simulink model "gm_broadwayIPC_2024b_interface"  (R2024b)
settings: Solver=FixedStepDiscrete  StartTime=0.0  StopTime=2  RelTol=1e-3  EnableMultiTasking=on
undefined symbols (not defined in the file or in its folder): gray
libraries: hdlsllib x20, visionhdlio x6, visionsources x2
Description:
  | Sobel Edge Detection Using the MATLAB(R) Function Block
  | This example shows how to use HDL Coder(TM) to check,
  | generate, and verify HDL code for a Sobel Edge Detection
  | block built using the MATLAB Function block.
settings Model: Creator=The MathWorks, Inc.  LastModifiedBy=Chris
settings SolverCC: AlgebraicLoopSolver=TrustRegion  PositivePriorityOrder=on
settings DataIOCC: LimitDataPoints=on  SaveFormat=Array  SignalLogging=off  ReturnWorkspaceOutputs=off
settings OptimizationCC: BlockReduction=off  ConditionallyExecuteInputs=off  EnhancedBackFolding=on  PassReuseOutputArgsAs=Individual arguments  ExpressionDepthLimit=2147483647  ZeroExternalMemoryAtStartup=off  ZeroInternalMemoryAtStartup=off  InitFltsAndDblsToZero=on  EfficientMapNaN2IntZero=off  MaxStackSize=64  OptimizeBlockOrder=speed  DifferentSizesBufferReuse=on  OptimizationCustomize=off  EfficientTunableParamExpr=on
settings DebuggingCC: AlgebraicLoopMsg=error  SaveWithParameterizedLinksMsg=none  UnderspecifiedInitializationDetection=Classic  MergeDetectMultiDrivingBlocksExec=none  SignalResolutionControl=TryResolveAllWithWarning  SingleTaskRateTransMsg=error  IntegerOverflowMsg=none  ParameterPrecisionLossMsg=none  ParameterTunabilityLossMsg=error  FcnCallInpInsideContextMsg=warning  UnconnectedInputMsg=warning  UnconnectedOutputMsg=warning  UnconnectedLineMsg=warning  AllowSymbolicDim=off  StateNameClashWarn=warning  StrictBusMsg=ErrorOnBusTreatedAsVector  SFUnexpectedBacktrackingDiag=warning  SFNoUnconditionalDefaultTransitionDiag=warning  SFExecutionAtInitializationDiag=none  IntegerSaturationMsg=none  ArithmeticOperatorsInVariantConditions=warning
settings HardwareCC: ProdBitPerPointer=32  ProdBitPerSizeT=32  ProdBitPerPtrDiffT=32  ProdLargestAtomicInteger=Long  ProdLargestAtomicFloat=Double  ProdWordSize=32  ProdLongLongMode=on  ProdHWDeviceType=ARM Compatible->ARM Cortex-A (32-bit)  TargetHWDeviceType=32-bit Generic
settings ModelReferenceCC: EnableRefExpFcnMdlSchedulingChecks=on  ModelReferenceNumInstancesAllowed=Single  PropagateSignalLabelsOutOfModel=off
settings SFSimCC: SimUseLocalCustomCode=off  MATLABDynamicMemAlloc=off  CustomCodeUndefinedFunction=UseInterfaceOnly
settings RTWCC: Description=Embedded Coder  SystemTargetFile=ert.tlc  HardwareBoard=Xilinx Zynq-7000 based board  TLCOptions="-aInlineSetEventsForThisBaseRateFcn=TLC_FALSE -aSuppressMultiTaskScheduler=TLC_FALSE  -aRateBasedStepFcn=0"  TemplateMakefile=ert_default_tmf  RTWUseLocalCustomCode=off  Toolchain=Linaro AArch32 Linux v6.3.1  GPUComputeCapability=3.5  DLArmComputeVersion=19.05
settings CodeAppCC: ForceParamTrailComments=on  IgnoreCustomStorageClasses=off  OperatorAnnotations=on  SimulinkDataObjDesc=on  SFDataObjDesc=on  InsertBlockDesc=on
settings ERTTargetCC: InlinedParameterPlacement=Hierarchical
settings ConfigComp: CovMetricSettings=dw  CovSaveCumulativeToWorkspaceVar=on  CovSaveSingleToWorkspaceVar=on  CovExternalEMLEnable=off

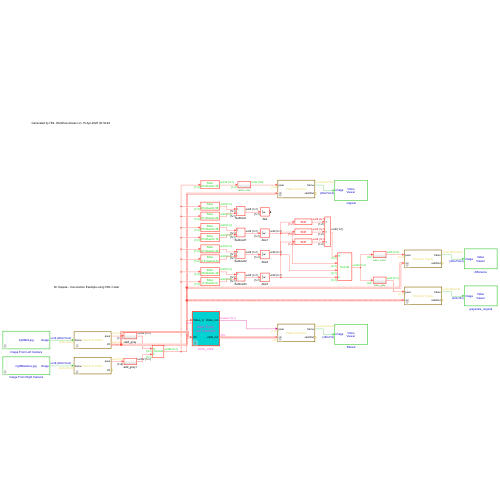
[thumbnail: Simulink's stored preview of the top-level diagram]
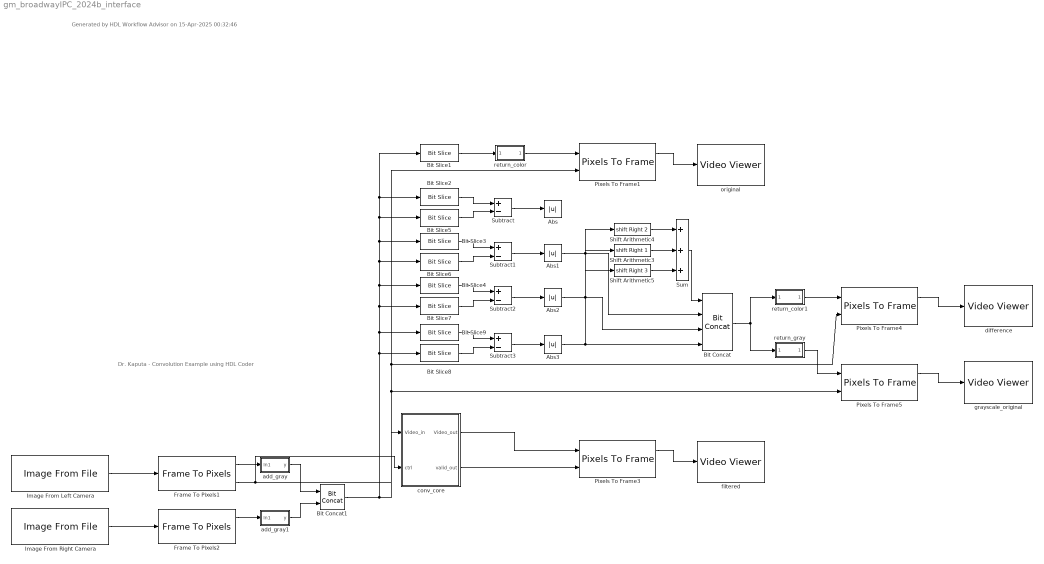
== system gm_broadwayIPC_2024b_interface ==
  note: Dr. Kaputa - Convolution Example using HDL Coder
  note: Generated by HDL Workflow Advisor on 15-Apr-2025 00:32:46
  Abs{,1..3} (4 alike) : Abs  OutDataTypeStr=uint8
  Bit Concat : hdlsllib/Logic and Bit Operations/Bit Concat  numInputs=4
  Bit Concat1 : hdlsllib/Logic and Bit Operations/Bit Concat  numInputs=2
  Bit Slice1 : hdlsllib/Logic and Bit Operations/Bit Slice  lidx=63  ridx=32
  Bit Slice2 : hdlsllib/Logic and Bit Operations/Bit Slice  lidx=63  ridx=56
  Bit Slice3 : hdlsllib/Logic and Bit Operations/Bit Slice  lidx=55  ridx=48
  Bit Slice4 : hdlsllib/Logic and Bit Operations/Bit Slice  lidx=47  ridx=40
  Bit Slice5 : hdlsllib/Logic and Bit Operations/Bit Slice  lidx=31  ridx=24
  Bit Slice6 : hdlsllib/Logic and Bit Operations/Bit Slice  lidx=23  ridx=16
  Bit Slice7 : hdlsllib/Logic and Bit Operations/Bit Slice  lidx=15  ridx=8
  Bit Slice8 : hdlsllib/Logic and Bit Operations/Bit Slice  lidx=7  ridx=0
  Bit Slice9 : hdlsllib/Logic and Bit Operations/Bit Slice  lidx=39  ridx=32
  Frame To Pixels1 : visionhdlio/Frame To Pixels  NumComponents=3  NumPixels=1  VideoFormat=Custom  ActivePixelsPerLine=R  ActiveVideoLines=C  TotalPixelsPerLine=R  TotalVideoLines=C  StartingActiveLine=1  FrontPorch=0  SampleTime=0  VideoFormatCache=Custom  ActivePixelsPerLineCache=R  ActiveVideoLinesCache=C  TotalPixelsPerLineCache=R  TotalVideoLinesCache=C  StartingActiveLineCache=1  FrontPorchCache=0
  Frame To Pixels2 : visionhdlio/Frame To Pixels  NumComponents=3  NumPixels=1  VideoFormat=Custom  ActivePixelsPerLine=R  ActiveVideoLines=C  TotalPixelsPerLine=R  TotalVideoLines=C  StartingActiveLine=1  FrontPorch=0  SampleTime=0  VideoFormatCache=Custom  ActivePixelsPerLineCache=R  ActiveVideoLinesCache=C  TotalPixelsPerLineCache=R  TotalVideoLinesCache=C  StartingActiveLineCache=1  FrontPorchCache=0
  Image From Left Camera : visionsources/Image From File  Tag=vipblks_nd  FileName=C:\Users\Chris\Documents\Repos\WiiSports\TennisTracker\BoradwaySimulink\rightBall.jpg  Ts=1  imagePorts=One multidimensional signal  OutPortLabels=R|G|B  ImageDataType=Inherit from input image  sdImageDataType=uint(8)  Signed=on  WordLength=16  FractionLengthMode=User-defined  FractionLength=15
  Image From Right Camera : visionsources/Image From File  Tag=vipblks_nd  FileName=C:\Users\Chris\Documents\Repos\WiiSports\TennisTracker\BoradwaySimulink\rightBaseline.jpg  Ts=1  imagePorts=One multidimensional signal  OutPortLabels=R|G|B  ImageDataType=Inherit from input image  sdImageDataType=uint(8)  Signed=on  WordLength=16  FractionLengthMode=User-defined  FractionLength=15
  Pixels To Frame1 : visionhdlio/Pixels To Frame  NumComponents=3  NumPixels=1  VideoFormat=Custom  ActivePixelsPerLine=R  ActiveVideoLines=C  TotalPixelsPerLine=R  TotalVideoLines=C  VideoFormatCache=Custom  ActivePixelsPerLineCache=R  ActiveVideoLinesCache=C  TotalPixelsPerLineCache=R  TotalVideoLinesCache=C
  Pixels To Frame3 : visionhdlio/Pixels To Frame  NumComponents=1  NumPixels=1  VideoFormat=Custom  ActivePixelsPerLine=R  ActiveVideoLines=C  TotalPixelsPerLine=R  TotalVideoLines=C  VideoFormatCache=Custom  ActivePixelsPerLineCache=R  ActiveVideoLinesCache=C  TotalPixelsPerLineCache=R  TotalVideoLinesCache=C
  Pixels To Frame4 : visionhdlio/Pixels To Frame  NumComponents=3  NumPixels=1  VideoFormat=Custom  ActivePixelsPerLine=R  ActiveVideoLines=C  TotalPixelsPerLine=R  TotalVideoLines=C  VideoFormatCache=Custom  ActivePixelsPerLineCache=R  ActiveVideoLinesCache=C  TotalPixelsPerLineCache=R  TotalVideoLinesCache=C
  Pixels To Frame5 : visionhdlio/Pixels To Frame  NumComponents=1  NumPixels=1  VideoFormat=Custom  ActivePixelsPerLine=R  ActiveVideoLines=C  TotalPixelsPerLine=R  TotalVideoLines=C  VideoFormatCache=Custom  ActivePixelsPerLineCache=R  ActiveVideoLinesCache=C  TotalPixelsPerLineCache=R  TotalVideoLinesCache=C
  Shift Arithmetic3 : ArithShift  BitShiftNumber=1  BitShiftDirection=Right
  Shift Arithmetic4 : ArithShift  BitShiftNumber=2  BitShiftDirection=Right
  Shift Arithmetic5 : ArithShift  BitShiftNumber=3  BitShiftDirection=Right
  Subtract{,1..3} (4 alike) : Sum  Inputs=+-
  Sum : Sum  Inputs=+++  OutDataTypeStr=uint8
  add_gray : Subsystem
  add_gray1 : Subsystem
  conv_core : Subsystem  TreatAsAtomicUnit=on  mask(AXI4-Lite/AXI4 Interface){}
      mask help:
      | This is an automatically generated subsystem block.
      | This contains the AXI interface blocks that communicate with the conv_core_ip IPCore generated from broadwayIPC_2024b/conv_core subsystem.
      mask Display: disp(sprintf('Xilinx Zynq \nAXI Interface'));
  difference : VideoViewer  FigPos=[994 1078 927 429]
  filtered : VideoViewer  colormapValue=gray(256)  FigPos=[66 1078 927 429]
  grayscale_original : VideoViewer  FigPos=[65 538 927 429]
  original : VideoViewer  FigPos=[995 538 927 429]
  return_color : Subsystem
  return_color1 : Subsystem
  return_gray : Subsystem
  wires:
  Bit Concat/1 -> return_color1/1(RGB), return_gray/1(RGB)
  Sum/1 -> Bit Concat/1
  Abs1/1 -> Bit Concat/2, Shift Arithmetic4/1
  Abs2/1 -> Bit Concat/3, Shift Arithmetic3/1
  Abs3/1 -> Bit Concat/4, Shift Arithmetic5/1
  Shift Arithmetic4/1 -> Sum/1
  Shift Arithmetic3/1 -> Sum/2
  Shift Arithmetic5/1 -> Sum/3
  return_gray/1(RGBVector) -> Pixels To Frame5/1
  Pixels To Frame5/1 -> grayscale_original/1
  Bit Slice8/1 -> Subtract3/2
  Bit Slice9/1 -> Subtract3/1
  Bit Slice7/1 -> Subtract2/2
  Bit Slice4/1 -> Subtract2/1
  Bit Slice6/1 -> Subtract1/2
  Bit Slice3/1 -> Subtract1/1
  Bit Slice5/1 -> Subtract/2
  Bit Slice2/1 -> Subtract/1
  Subtract3/1 -> Abs3/1
  Subtract2/1 -> Abs2/1
  Subtract1/1 -> Abs1/1
  return_color1/1(RGBVector) -> Pixels To Frame4/1
  Subtract/1 -> Abs/1
  Pixels To Frame4/1 -> difference/1
  Bit Slice1/1 -> return_color/1(RGB)
  add_gray1/1(y) -> Bit Concat1/2
  add_gray/1(y) -> Bit Concat1/1
  Frame To Pixels2/1 -> add_gray1/1(In1)
  Frame To Pixels1/2 -> Pixels To Frame4/2, Pixels To Frame1/2, Pixels To Frame5/2, conv_core/2(ctrl)
  Image From Right Camera/1 -> Frame To Pixels2/1
  conv_core/1(Video_out) -> Pixels To Frame3/1
  Bit Concat1/1 -> Bit Slice2/1, Bit Slice1/1, Bit Slice5/1, Bit Slice3/1, Bit Slice6/1, Bit Slice4/1, Bit Slice7/1, Bit Slice9/1, Bit Slice8/1, conv_core/1(Video_in)
  conv_core/2(valid_out) -> Pixels To Frame3/2
  Pixels To Frame3/1 -> filtered/1
  Frame To Pixels1/1 -> add_gray/1(In1)
  return_color/1(RGBVector) -> Pixels To Frame1/1
  Pixels To Frame1/1 -> original/1
  Image From Left Camera/1 -> Frame To Pixels1/1

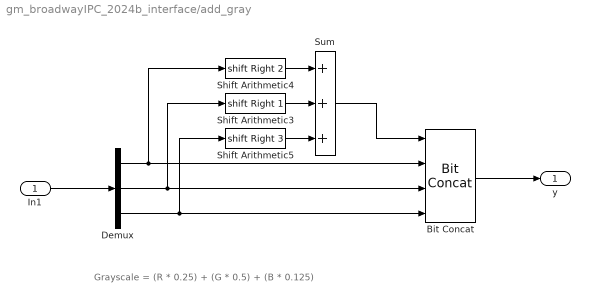
== system gm_broadwayIPC_2024b_interface/add_gray ==
  note: Grayscale = (R * 0.25) + (G * 0.5) + (B * 0.125)
  In1 : Inport
  Bit Concat : hdlsllib/Logic and Bit Operations/Bit Concat  numInputs=4
  Demux : Demux  Outputs=3
  Shift Arithmetic3 : ArithShift  BitShiftNumber=1  BitShiftDirection=Right
  Shift Arithmetic4 : ArithShift  BitShiftNumber=2  BitShiftDirection=Right
  Shift Arithmetic5 : ArithShift  BitShiftNumber=3  BitShiftDirection=Right
  Sum : Sum  Inputs=+++  OutDataTypeStr=uint8
  y : Outport
  wires:
  Shift Arithmetic5/1 -> Sum/3
  Shift Arithmetic3/1 -> Sum/2
  Shift Arithmetic4/1 -> Sum/1
  Sum/1 -> Bit Concat/1
  Demux/3 -> Bit Concat/4, Shift Arithmetic5/1
  Demux/1 -> Bit Concat/2, Shift Arithmetic4/1
  Demux/2 -> Bit Concat/3, Shift Arithmetic3/1
  In1/1 -> Demux/1
  Bit Concat/1 -> y/1

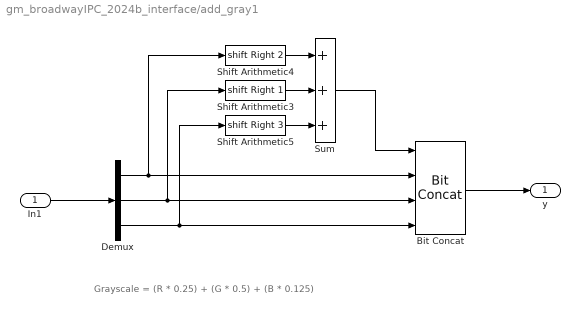
== system gm_broadwayIPC_2024b_interface/add_gray1 ==
  note: Grayscale = (R * 0.25) + (G * 0.5) + (B * 0.125)
  In1 : Inport
  Bit Concat : hdlsllib/Logic and Bit Operations/Bit Concat  numInputs=4
  Demux : Demux  Outputs=3
  Shift Arithmetic3 : ArithShift  BitShiftNumber=1  BitShiftDirection=Right
  Shift Arithmetic4 : ArithShift  BitShiftNumber=2  BitShiftDirection=Right
  Shift Arithmetic5 : ArithShift  BitShiftNumber=3  BitShiftDirection=Right
  Sum : Sum  Inputs=+++  OutDataTypeStr=uint8
  y : Outport
  wires:
  Sum/1 -> Bit Concat/1
  Shift Arithmetic5/1 -> Sum/3
  Shift Arithmetic3/1 -> Sum/2
  Shift Arithmetic4/1 -> Sum/1
  Demux/3 -> Bit Concat/4, Shift Arithmetic5/1
  Demux/1 -> Bit Concat/2, Shift Arithmetic4/1
  Demux/2 -> Bit Concat/3, Shift Arithmetic3/1
  In1/1 -> Demux/1
  Bit Concat/1 -> y/1

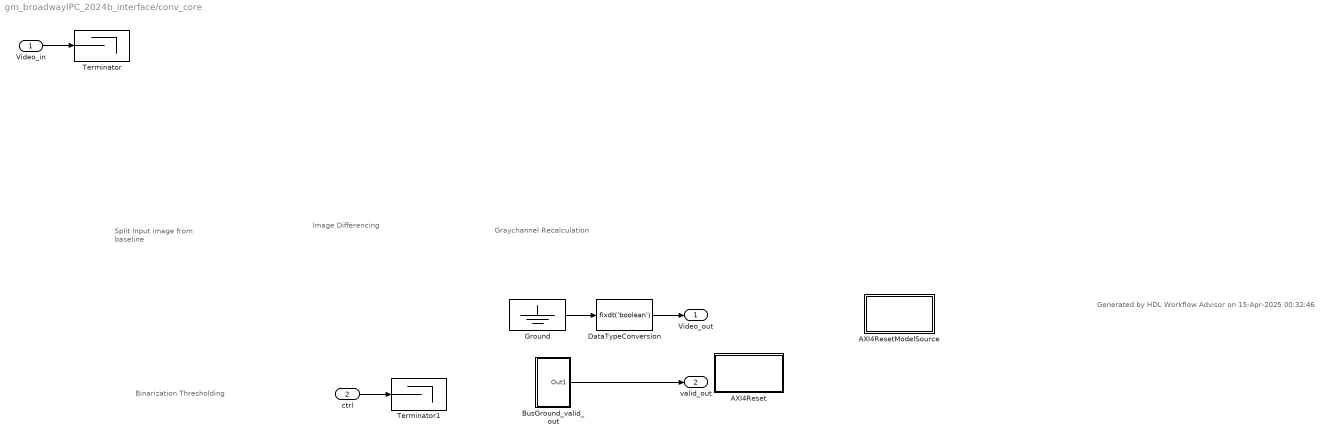
== system gm_broadwayIPC_2024b_interface/conv_core ==
  note: Binarization Thresholding
  note: Image
      | Differencing
  note: Split Input image
      | from baseline
  note: Graychannel Recalculation
  note: Generated by HDL Workflow Advisor on 15-Apr-2025 00:32:46
  Video_in : Inport
  ctrl : Inport  Port=2
  AXI4Reset : Subsystem  mask(System Start){ShowInLibBrowser=0}
      mask prompts: ShowInLibBrowser "Simulink:masks:CustCodeMaskParam1_MP"
      settings: CopyFcn=cccopyfcn(gcb)  OpenFcn=ccopenfcn('System Start Function')
      mask Help: eval('feval(''rtwprivate'',''rtwhelpview'',''rtw_sys_start_block'')');
      mask Display: disp('System\nStart');
  AXI4ResetModelSource : Subsystem  mask(Model Source){ShowInLibBrowser=0}
      mask prompts: ShowInLibBrowser "Simulink:masks:CustCodeMaskParam1_MP"
      settings: CopyFcn=cccopyfcn(gcb)  OpenFcn=ccopenfcn('Model Source')
      mask Help: eval('feval(''rtwprivate'',''rtwhelpview'',''rtw_model_source_block'')');
      mask Display: disp('Model\nSource');
  BusGround_valid_out : Subsystem
  DataTypeConversion : DataTypeConversion  OutDataTypeStr=fixdt('boolean')  ConvertRealWorld=Stored Integer (SI)  SaturateOnIntegerOverflow=off  RndMeth=Floor
  Ground : Ground
  Terminator : Terminator
  Terminator1 : Terminator
  Video_out : Outport  VectorParamsAs1DForOutWhenUnconnected=off
  valid_out : Outport  Port=2  VectorParamsAs1DForOutWhenUnconnected=off
  wires:
  Video_in/1 -> Terminator/1
  ctrl/1 -> Terminator1/1
  DataTypeConversion/1 -> Video_out/1
  Ground/1 -> DataTypeConversion/1
  BusGround_valid_out/1(Out1) -> valid_out/1

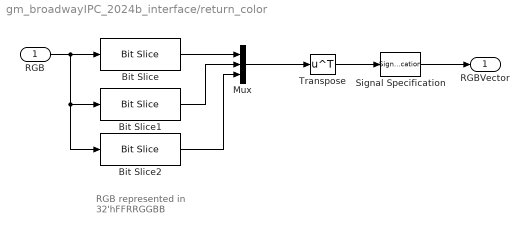
== system gm_broadwayIPC_2024b_interface/return_color ==
  note: RGB represented in
      | 32'hFFRRGGBB
  RGB : Inport
  Bit Slice : hdlsllib/Logic and Bit Operations/Bit Slice  lidx=23  ridx=16
  Bit Slice1 : hdlsllib/Logic and Bit Operations/Bit Slice  lidx=15  ridx=8
  Bit Slice2 : hdlsllib/Logic and Bit Operations/Bit Slice  lidx=7  ridx=0
  Mux : Mux  Inputs=3
  Signal Specification : SignalSpecification
  Transpose : Math  Operator=transpose  SignedPower=on
  RGBVector : Outport  VectorParamsAs1DForOutWhenUnconnected=off
  wires:
  Mux/1 -> Transpose/1
  Bit Slice/1 -> Mux/1
  Bit Slice2/1 -> Mux/3
  Bit Slice1/1 -> Mux/2
  RGB/1 -> Bit Slice2/1, Bit Slice1/1, Bit Slice/1
  Transpose/1 -> Signal Specification/1
  Signal Specification/1 -> RGBVector/1

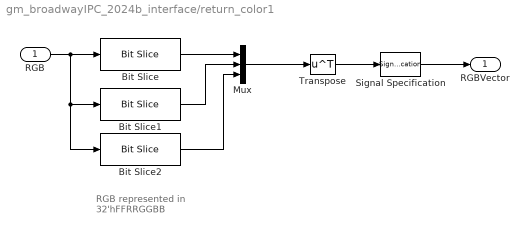
== system gm_broadwayIPC_2024b_interface/return_color1 ==
  note: RGB represented in
      | 32'hFFRRGGBB
  RGB : Inport
  Bit Slice : hdlsllib/Logic and Bit Operations/Bit Slice  lidx=23  ridx=16
  Bit Slice1 : hdlsllib/Logic and Bit Operations/Bit Slice  lidx=15  ridx=8
  Bit Slice2 : hdlsllib/Logic and Bit Operations/Bit Slice  lidx=7  ridx=0
  Mux : Mux  Inputs=3
  Signal Specification : SignalSpecification
  Transpose : Math  Operator=transpose  SignedPower=on
  RGBVector : Outport  VectorParamsAs1DForOutWhenUnconnected=off
  wires:
  Mux/1 -> Transpose/1
  Bit Slice/1 -> Mux/1
  Bit Slice2/1 -> Mux/3
  Bit Slice1/1 -> Mux/2
  RGB/1 -> Bit Slice2/1, Bit Slice1/1, Bit Slice/1
  Transpose/1 -> Signal Specification/1
  Signal Specification/1 -> RGBVector/1

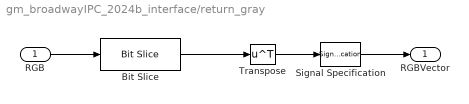
== system gm_broadwayIPC_2024b_interface/return_gray ==
  RGB : Inport
  Bit Slice : hdlsllib/Logic and Bit Operations/Bit Slice  lidx=31  ridx=24
  Signal Specification : SignalSpecification
  Transpose : Math  Operator=transpose  SignedPower=on
  RGBVector : Outport  VectorParamsAs1DForOutWhenUnconnected=off
  wires:
  Bit Slice/1 -> Transpose/1
  Signal Specification/1 -> RGBVector/1
  Transpose/1 -> Signal Specification/1
  RGB/1 -> Bit Slice/1

== system gm_broadwayIPC_2024b_interface/conv_core/AXI4Reset ==

== system gm_broadwayIPC_2024b_interface/conv_core/AXI4ResetModelSource ==

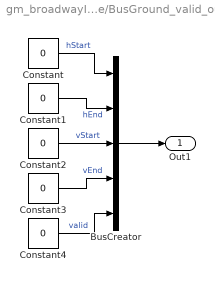
== system gm_broadwayIPC_2024b_interface/conv_core/BusGround_valid_out ==
  BusCreator : BusCreator  Inputs=5
  Constant{,1..4} (5 alike) : Constant  Value=0  OutDataTypeStr=fixdt('boolean')  SampleTime=-1
  Out1 : Outport
  wires:
  Constant3/1 -> BusCreator/4  "vEnd"
  Constant2/1 -> BusCreator/3  "vStart"
  Constant/1 -> BusCreator/1  "hStart"
  Constant1/1 -> BusCreator/2  "hEnd"
  Constant4/1 -> BusCreator/5  "valid"
  BusCreator/1 -> Out1/1
